simulink model "simulinkmodel"  (R2020a)
settings: Solver=VariableStepAuto  StartTime=0.0  StopTime=10.0  RelTol=1e-3
values from neighbouring files (symbols this model uses):
  g = 9.81    [Systemmodeling.m]
  kd = 2*zeta*wn/K_bb    [Systemmodeling.m]
  kp = wn^2/K_bb    [Systemmodeling.m]
  Lt = .275    (= 0.275)    [Systemmodeling.m]
  Ltc = Lt*100    (= 27.5)    [Systemmodeling.m]
  px = 140    [Systemmodeling.m]
  py = 190    [Systemmodeling.m]
  rarm = .0254    (= 0.0254)    [Systemmodeling.m]
  res = 200    [Systemmodeling.m]
settings Model: Creator=mx13m  LastModifiedBy=mx13m

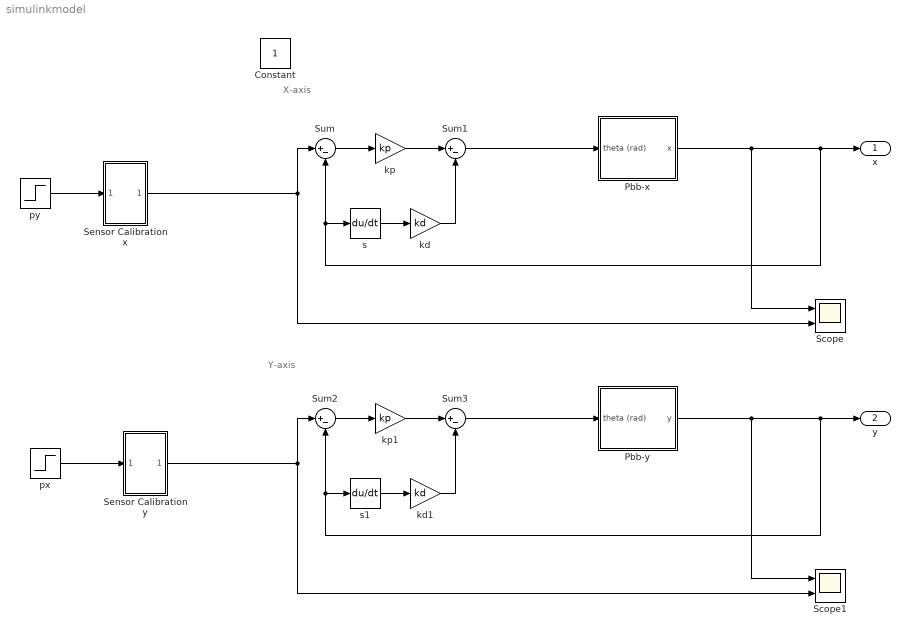
== system simulinkmodel ==
  note: Y-axis
  note: X-axis
  Pbb-x : Subsystem
  Pbb-y : Subsystem
  Scope : Scope  NumInputPorts=2
  Scope1 : Scope  NumInputPorts=2
  Sensor Calibration x : Subsystem
  Sensor Calibration y : Subsystem
  Sum{,1..3} (4 alike) : Sum  Inputs=|+-
  kd : Gain  Gain=kd
  kd1 : Gain  Gain=kd
  kp : Gain  Gain=kp
  kp1 : Gain  Gain=kp
  px : Step  Time=0  After=px  SampleTime=0
  py : Step  Time=0  After=py  SampleTime=0
  s : Derivative
  s1 : Derivative
  x : Outport
  y : Outport  Port=2
  Constant : Constant  IOType=siggen
  wires:
  s/1 -> kd/1
  kd/1 -> Sum1/2
  Sum/1 -> kp/1
  kp/1 -> Sum1/1
  Sum1/1 -> Pbb-x/1(theta (rad))
  Sum3/1 -> Pbb-y/1(theta (rad))
  kp1/1 -> Sum3/1
  Pbb-y/1(y) -> Scope1/1, Sum2/2, s1/1, y/1
  s1/1 -> kd1/1
  kd1/1 -> Sum3/2
  Sum2/1 -> kp1/1
  Pbb-x/1(x) -> Scope/1, Sum/2, s/1, x/1
  Sensor Calibration x/1(Out1) -> Sum/1, Scope/2
  py/1 -> Sensor Calibration x/1(In1)
  Sensor Calibration y/1(Out1) -> Sum2/1, Scope1/2
  px/1 -> Sensor Calibration y/1(In1)

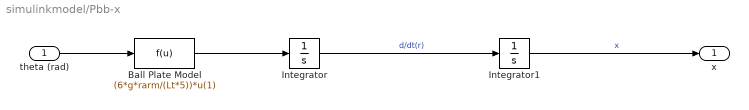
== system simulinkmodel/Pbb-x ==
  theta (rad) : Inport
  Ball Plate Model : Fcn  Expr=(6*g*rarm/(Lt*5))*u(1)
  Integrator : Integrator
  Integrator1 : Integrator
  x : Outport
  wires:
  Integrator1/1 -> x/1  "x"
  Ball Plate Model/1 -> Integrator/1
  theta (rad)/1 -> Ball Plate Model/1
  Integrator/1 -> Integrator1/1  "d/dt(r)"

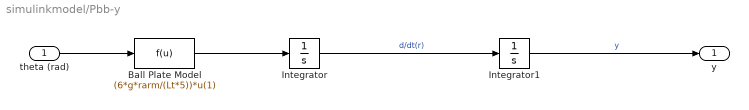
== system simulinkmodel/Pbb-y ==
  theta (rad) : Inport
  Ball Plate Model : Fcn  Expr=(6*g*rarm/(Lt*5))*u(1)
  Integrator : Integrator
  Integrator1 : Integrator
  y : Outport
  wires:
  Integrator1/1 -> y/1  "y"
  Ball Plate Model/1 -> Integrator/1
  theta (rad)/1 -> Ball Plate Model/1
  Integrator/1 -> Integrator1/1  "d/dt(r)"

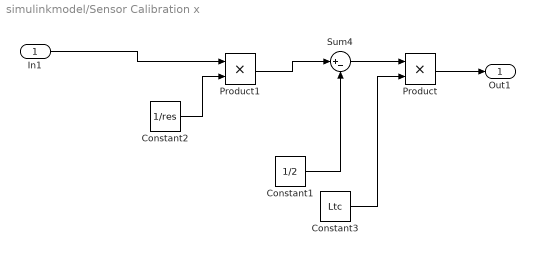
== system simulinkmodel/Sensor Calibration x ==
  In1 : Inport
  Constant1 : Constant  Value=1/2
  Constant2 : Constant  Value=1/res
  Constant3 : Constant  Value=Ltc
  Product : Product
  Product1 : Product
  Sum4 : Sum  Inputs=|+-
  Out1 : Outport
  wires:
  Constant3/1 -> Product/2
  In1/1 -> Product1/1
  Constant2/1 -> Product1/2
  Product1/1 -> Sum4/1
  Constant1/1 -> Sum4/2
  Sum4/1 -> Product/1
  Product/1 -> Out1/1

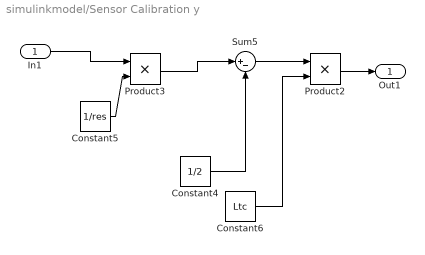
== system simulinkmodel/Sensor Calibration y ==
  In1 : Inport
  Constant4 : Constant  Value=1/2
  Constant5 : Constant  Value=1/res
  Constant6 : Constant  Value=Ltc
  Product2 : Product
  Product3 : Product
  Sum5 : Sum  Inputs=|+-
  Out1 : Outport
  wires:
  Product2/1 -> Out1/1
  Constant6/1 -> Product2/2
  Product3/1 -> Sum5/1
  In1/1 -> Product3/1
  Sum5/1 -> Product2/1
  Constant5/1 -> Product3/2
  Constant4/1 -> Sum5/2
